simulink model "signal_conversion"  (R2020b)
settings: Solver=FixedStepAuto  StartTime=0.0  StopTime=stop_time  RelTol=1e-3
settings Model: Creator=conno  LastModifiedBy=conno
settings DataIOCC: ReturnWorkspaceOutputs=off
settings OptimizationCC: DefaultParameterBehavior=Inlined

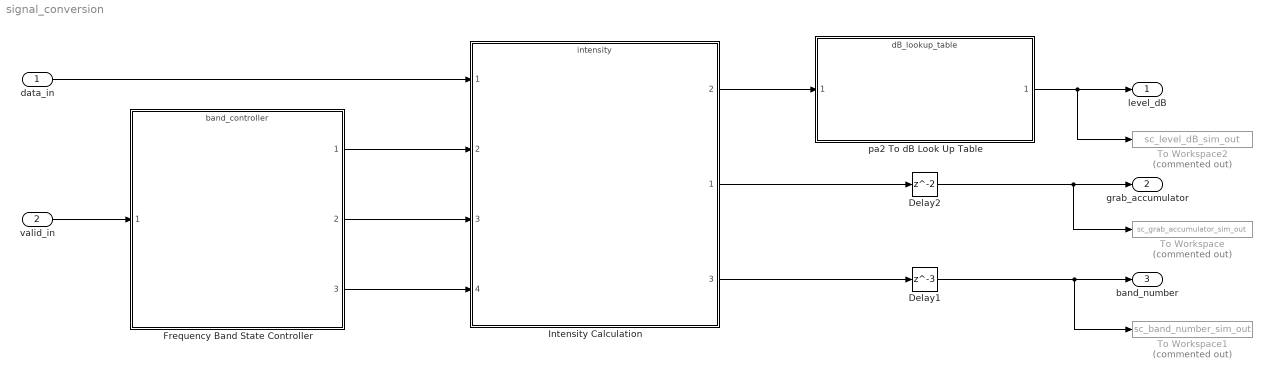
== system signal_conversion ==
  data_in : Inport
  valid_in : Inport  Port=2  OutDataTypeStr=boolean
  Delay1 : Delay  DelayLength=3  InitialCondition=0
  Delay2 : Delay  InitialCondition=0
  Frequency Band State Controller : ModelReference  ModelNameDialog=band_controller.slx  SimulationMode=Normal  ModelReferenceVersion=2.51
  Intensity Calculation : ModelReference  ModelNameDialog=intensity.slx  SimulationMode=Normal  ModelReferenceVersion=2.48
      settings: PortSchema="{\"entries\":[{\"content\":{\"sides\":[{\"content\":{\"connectorIds\":[\"In1\",\"In2\",\"In3\",\"In4\"]},\"type\":\"ConnectorPlacement.EquallySpacedRectSide\",\"uuid\":\"1715ac82-9bf9-45f0-89dd-ef254743e0d0\"},{\"content\":{\"connectorIds\":[\"Out2\",\"Out1\",\"Out3\"],\"side\":\"RIGHT\"},\"type\":\"ConnectorPlacement.EquallySpacedRectSide\",\"uuid\":\"1ac9df1c-3178-4a7b-9102-20b65dc3805c\"},{\"content\":{\"connectorIds\":[],\"side\":\"TOP\"},\"type\":\"ConnectorPlacement.EquallySpacedRectSide\",\"uuid\":\"25569bb4-aab4-4363-9b28-b47c18a3e185\"},{\"content\":{\"connectorIds\":[],\"side\":\"HIDDEN\"},\"type\":\"ConnectorPlacement.EquallySpacedRectSide\",\"uuid\":\"29078c1d-30f1-4610-ae90-b869cbef1c5f\"}]},\"type\":\"ConnectorPlacement.EquallySpacedConnector\",\"uuid\":\"9fe03e1d-ee03-41fe-8a8f-68791f98f5c0\"}],\"packageUris\":[\"http://schema.mathworks.com/mf0/Connector/R2020b\"],\"version\":\"1.0\"}"
  To Workspace : ToWorkspace  Commented=on  VariableName=sc_grab_accumulator_sim_out  SampleTime=-1
  To Workspace1 : ToWorkspace  Commented=on  VariableName=sc_band_number_sim_out  SampleTime=-1
  To Workspace2 : ToWorkspace  Commented=on  VariableName=sc_level_dB_sim_out  SampleTime=-1
  pa2 To dB Look Up Table : ModelReference  ModelNameDialog=dB_lookup_table.slx  SimulationMode=Normal  ModelReferenceVersion=2.47
  level_dB : Outport
  grab_accumulator : Outport  Port=2
  band_number : Outport  Port=3
  wires:
  pa2 To dB Look Up Table/1 -> To Workspace2/1, level_dB/1
  Intensity Calculation/2 -> pa2 To dB Look Up Table/1
  Intensity Calculation/1 -> Delay2/1
  Intensity Calculation/3 -> Delay1/1
  Frequency Band State Controller/1 -> Intensity Calculation/2
  Frequency Band State Controller/2 -> Intensity Calculation/3
  Frequency Band State Controller/3 -> Intensity Calculation/4
  valid_in/1 -> Frequency Band State Controller/1
  data_in/1 -> Intensity Calculation/1
  Delay2/1 -> To Workspace/1, grab_accumulator/1
  Delay1/1 -> To Workspace1/1, band_number/1
